simulink model "a2024_V2X_6V_Simulink_model"  (R2023b)
settings: Solver=VariableStepAuto  StartTime=0.0  StopTime=30  MaxStep=1e-2  RelTol=1e-3  AbsTol=1e-3
values from neighbouring files (symbols this model uses):
  b = 1.6    [a2024_v2x_matlab_6veh.m]
  mEgo = 1500    [a2024_v2x_matlab_6veh.m]
  Mode = 1    [a2024_v2x_matlab_6veh.m]    (also in v2x_matlab.m; v2x_matlabV2.m; v2x_matlab_6veh.m; v2x_matlab_R.m)
  pilot = (randi(s,[0 1],pilotsPerSym,1)-0.5)*2    [v2x_matlab.m]
  RxPowerV1 = zeros(sizeEgoWP+2, sizeV1WP+2)    [a2024_v2x_matlab_6veh.m]
  RxPowerV2 = zeros(sizeEgoWP+2, sizeV2WP+2)    [a2024_v2x_matlab_6veh.m]
  RxPowerV3 = zeros(sizeEgoWP+2, sizeV3WP+2)    [a2024_v2x_matlab_6veh.m]
  RxPowerV4 = zeros(sizeEgoWP+2, sizeV4WP+2)    [a2024_v2x_matlab_6veh.m]
  RxPowerV5 = zeros(sizeEgoWP+2, sizeV5WP+2)    [a2024_v2x_matlab_6veh.m]
  RxPowerV6 = zeros(sizeEgoWP+2, sizeV6WP+2)    [a2024_v2x_matlab_6veh.m]
  sampleTime = 0.1    [a2024_v2x_matlab_6veh.m]    (also in v2x_matlab.m; v2x_matlabV2.m; v2x_matlab_6veh.m; v2x_matlab_R.m)
  t_gap = 1.4    [a2024_v2x_matlab_6veh.m]
  waypoints = [egoWP(:,2) egoWP(:,1), zeroforwp]    [a2024_v2x_matlab_6veh.m]    (also in misc.m = data.data.ActorSpecifications(1,1).Waypoints(:,[1,2]); v2x_matlab.m = data.data.ActorSpecifications(1,1).Waypoints(:,[1,2]); v2x_matlabV2.m = [5 -1.6 0; v2x_matlab_R.m = [5 -1.6 0)
  ZeroActors = struct(     'ActorID',0,     'Position', [1000 1000 1000],      'Velocity', [0 0 0],      'Roll', 0,      'Pitch', 0,      'Yaw', 0,      'AngularVelocity', [0 0 0])    [v2x_matlabV2.m]    (also in v2x_matlab_R.m)
undefined symbols (not defined in the file or in its folder): driving, PredictionHorizon, Ts
libraries: commofdm x50, commcnvcod2 x39, simulink x34, commdigbbndam3 x31, commblkintrlv2 x26, commdigbbndpm3 x14, simulink_extras x12, drivingscenarioandsensors x3, mpcadaslib x2, commchan3 x1, vehdynlibdriver x1, commrandsrc3 x1
(part 2 of 6)

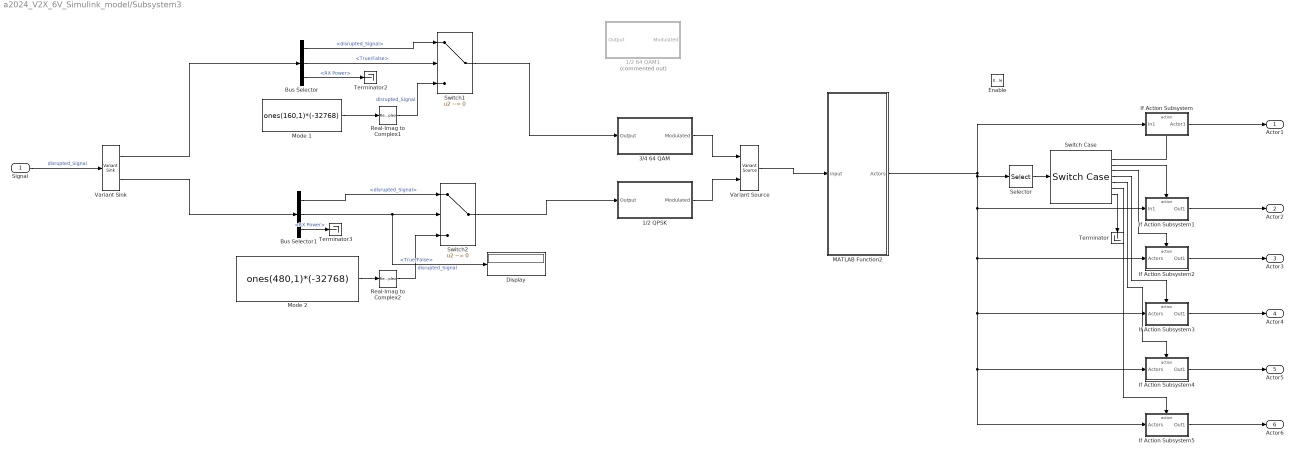
== system a2024_V2X_6V_Simulink_model/Subsystem3 ==
  Signal : Inport
  Enable : EnablePort
  1/2 64 QAM1 : Subsystem  Commented=on  TreatAsAtomicUnit=on
  1/2 QPSK : Subsystem  TreatAsAtomicUnit=on
  3/4 64 QAM : Subsystem  TreatAsAtomicUnit=on
  Bus Selector : BusSelector  OutputSignals=disrupted_Signal,True/False,RX Power
  Bus Selector1 : BusSelector  OutputSignals=disrupted_Signal,True/False,RX Power
  Display : Display
  If Action Subsystem : Subsystem  TreatAsAtomicUnit=on
  If Action Subsystem1 : Subsystem  TreatAsAtomicUnit=on
  If Action Subsystem2 : Subsystem  TreatAsAtomicUnit=on
  If Action Subsystem3 : Subsystem  TreatAsAtomicUnit=on
  If Action Subsystem4 : Subsystem  TreatAsAtomicUnit=on
  If Action Subsystem5 : Subsystem  TreatAsAtomicUnit=on
  MATLAB Function2 : MATLAB Function  TreatAsAtomicUnit=on  SystemSampleTime=0.01
  Mode 1 : Constant  Value=ones(160,1)*(-32768)  OutDataTypeStr=Inherit: Inherit via back propagation
  Mode 2 : Constant  Value=ones(480,1)*(-32768)  OutDataTypeStr=Inherit: Inherit via back propagation
  Real-Imag to Complex1 : RealImagToComplex  Input=Real
  Real-Imag to Complex2 : RealImagToComplex  Input=Real
  Selector : Selector  IndexOptions=Index vector (dialog)  Indices=[3]  OutputSizes=1
  Switch Case : SwitchCase  CaseConditions={1,2,3,4,5,6}
  Switch1 : Switch  Criteria=u2 ~= 0  OutDataTypeStr=double  SaturateOnIntegerOverflow=off  InputSameDT=off
  Switch2 : Switch  Criteria=u2 ~= 0  OutDataTypeStr=double  SaturateOnIntegerOverflow=off  InputSameDT=off
  Terminator : Terminator
  Terminator2 : Terminator
  Terminator3 : Terminator
  Variant Sink : VariantSink
  Variant Source : VariantSource
  Actor1 : Outport
  Actor2 : Outport  Port=2
  Actor3 : Outport  Port=3
  Actor4 : Outport  Port=4
  Actor5 : Outport  Port=5
  Actor6 : Outport  Port=6
  wires:
  Selector/1 -> Switch Case/1
  Switch Case/1 -> If Action Subsystem/Action
  If Action Subsystem/1(Actor1) -> Actor1/1
  If Action Subsystem1/1(Out1) -> Actor2/1
  Switch Case/2 -> If Action Subsystem1/Action
  If Action Subsystem2/1(Out1) -> Actor3/1
  Switch Case/3 -> If Action Subsystem2/Action
  If Action Subsystem3/1(Out1) -> Actor4/1
  MATLAB Function2/1(Actors) -> If Action Subsystem5/1(Actors), If Action Subsystem4/1(Actors), If Action Subsystem3/1(Actors), If Action Subsystem2/1(Actors), If Action Subsystem1/1(In1), Selector/1, If Action Subsystem/1(In1)
  Switch Case/4 -> If Action Subsystem3/Action
  Switch Case/7 -> Terminator/1
  If Action Subsystem4/1(Out1) -> Actor5/1
  Switch Case/5 -> If Action Subsystem4/Action
  If Action Subsystem5/1(Out1) -> Actor6/1
  Switch Case/6 -> If Action Subsystem5/Action
  3/4 64 QAM/1(Modulated) -> Variant Source/1
  1/2 QPSK/1(Modulated) -> Variant Source/2
  Variant Source/1 -> MATLAB Function2/1(input)
  Switch1/1 -> 3/4 64 QAM/1(Output)
  Switch2/1 -> 1/2 QPSK/1(Output)
  Signal/1 -> Variant Sink/1  "disrupted_Signal"
  Variant Sink/1 -> Bus Selector/1
  Variant Sink/2 -> Bus Selector1/1
  Bus Selector/1 -> Switch1/1  "<disrupted_Signal>"
  Bus Selector/3 -> Terminator2/1  "<RX Power>"
  Bus Selector/2 -> Switch1/2  "<True/False>"
  Mode 1/1 -> Real-Imag to Complex1/1
  Real-Imag to Complex1/1 -> Switch1/3  "disrupted_Signal"
  Mode 2/1 -> Real-Imag to Complex2/1
  Bus Selector1/1 -> Switch2/1  "<disrupted_Signal>"
  Real-Imag to Complex2/1 -> Switch2/3  "disrupted_Signal"
  Bus Selector1/2 -> Display/1, Switch2/2  "<True/False>"
  Bus Selector1/3 -> Terminator3/1  "<RX Power>"

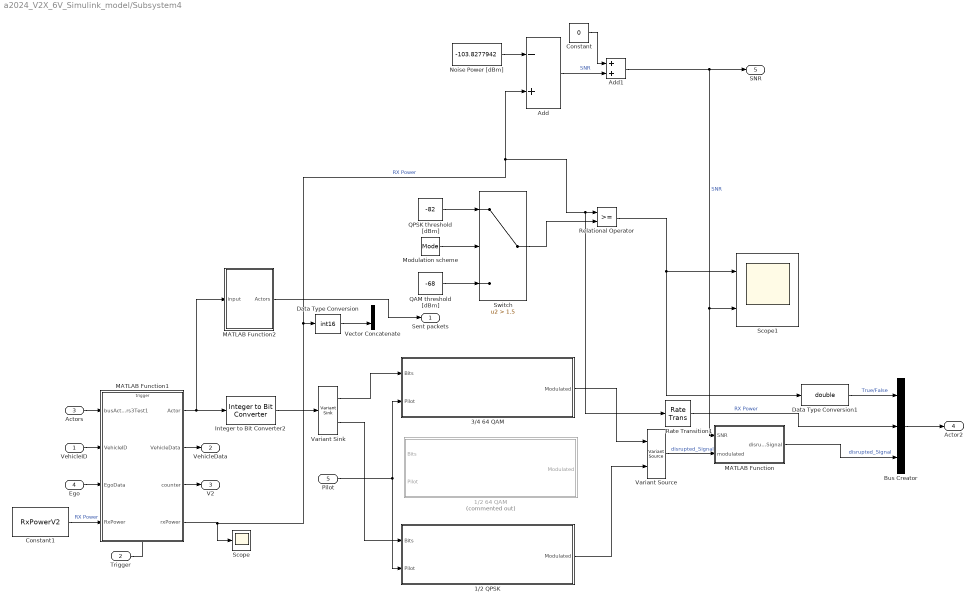
== system a2024_V2X_6V_Simulink_model/Subsystem4 ==
  VehicleID : Inport
  Trigger : Inport  Port=2
  Actors : Inport  Port=3
  Ego : Inport  Port=4
  Pilot : Inport  Port=5
  1/2 64 QAM : Subsystem  Commented=on  TreatAsAtomicUnit=on
  1/2 QPSK : Subsystem  TreatAsAtomicUnit=on
  3/4 64 QAM : Subsystem  TreatAsAtomicUnit=on
  Add : Sum  Inputs=-+
  Add1 : Sum
  Bus Creator : BusCreator  Inputs=3
  Constant : Constant  Value=0
  Constant1 : Constant  Value=RxPowerV2
  Data Type Conversion : DataTypeConversion  OutDataTypeStr=int16  SaturateOnIntegerOverflow=off  RndMeth=Floor
  Data Type Conversion1 : DataTypeConversion  OutDataTypeStr=double  SaturateOnIntegerOverflow=off  RndMeth=Floor
  Integer to Bit Converter2 : simulink/Logic and Bit Operations/Integer to Bit Converter  nbits=16  signedInputValues=Signed  bitOrder=MSB first  outDtype=boolean
  MATLAB Function : MATLAB Function  TreatAsAtomicUnit=on
  MATLAB Function1 : MATLAB Function  TreatAsAtomicUnit=on
  MATLAB Function2 : MATLAB Function  TreatAsAtomicUnit=on  SystemSampleTime=0.01
  Modulation scheme : Constant  Value=Mode
  Noise Power [dBm] : Constant  Value=-103.8277942
  QAM threshold [dBm] : Constant  Value=-68
  QPSK threshold [dBm] : Constant  Value=-82
  Rate Transition1 : RateTransition  OutPortSampleTime=sampleTime/10
  Relational Operator : RelationalOperator  OutDataTypeStr=boolean  RndMeth=Simplest  InputSameDT=off
  Scope : Scope
  Scope1 : Scope  NumInputPorts=2
  Switch : Switch  Criteria=u2 > Threshold  Threshold=1.5  SaturateOnIntegerOverflow=off  InputSameDT=off
  Variant Sink : VariantSink
  Variant Source : VariantSource
  Vector Concatenate : Concatenate
  Sent packets : Outport
  VehicleData : Outport  Port=2
  V2 : Outport  Port=3
  Actor2 : Outport  Port=4
  SNR : Outport  Port=5
  wires:
  Constant/1 -> Add1/1
  Add/1 -> Add1/2  "SNR"
  Variant Source/1 -> MATLAB Function/2(modulated)  "disrupted_Signal"
  Rate Transition1/1 -> Bus Creator/2  "RX Power"
  Data Type Conversion1/1 -> Bus Creator/1  "True/False"
  Data Type Conversion/1 -> Vector Concatenate/2
  MATLAB Function/1(disrupted_Signal) -> Bus Creator/3  "disrupted_Signal"
  MATLAB Function2/1(Actors) -> Sent packets/1
  Bus Creator/1 -> Actor2/1
  Constant1/1 -> MATLAB Function1/4(RxPower)  "RX Power"
  MATLAB Function1/4(rxPower) -> Add/2, Relational Operator/1, Rate Transition1/1, Data Type Conversion/1, Scope/1  "RX Power"
  Relational Operator/1 -> Scope1/1, Data Type Conversion1/1
  Switch/1 -> Relational Operator/2
  Add1/1 -> SNR/1, Scope1/2, MATLAB Function/1(SNR)  "SNR"
  Modulation scheme/1 -> Switch/2
  QAM threshold [dBm]/1 -> Switch/3
  QPSK threshold [dBm]/1 -> Switch/1
  Noise Power [dBm]/1 -> Add/1
  Variant Sink/2 -> 1/2 QPSK/1(Bits)
  Variant Sink/1 -> 3/4 64 QAM/1(Bits)
  1/2 QPSK/1(Modulated) -> Variant Source/2
  3/4 64 QAM/1(Modulated) -> Variant Source/1
  Pilot/1 -> 3/4 64 QAM/2(Pilot), 1/2 QPSK/2(Pilot)
  Integer to Bit Converter2/1 -> Variant Sink/1
  Trigger/1 -> MATLAB Function1/Trigger
  MATLAB Function1/3(counter) -> V2/1
  MATLAB Function1/2(VehicleData) -> VehicleData/1
  VehicleID/1 -> MATLAB Function1/2(VehicleID)
  Actors/1 -> MATLAB Function1/1(busActors3Test1)
  Ego/1 -> MATLAB Function1/3(EgoData)
  MATLAB Function1/1(Actor) -> Integer to Bit Converter2/1, MATLAB Function2/1(input)

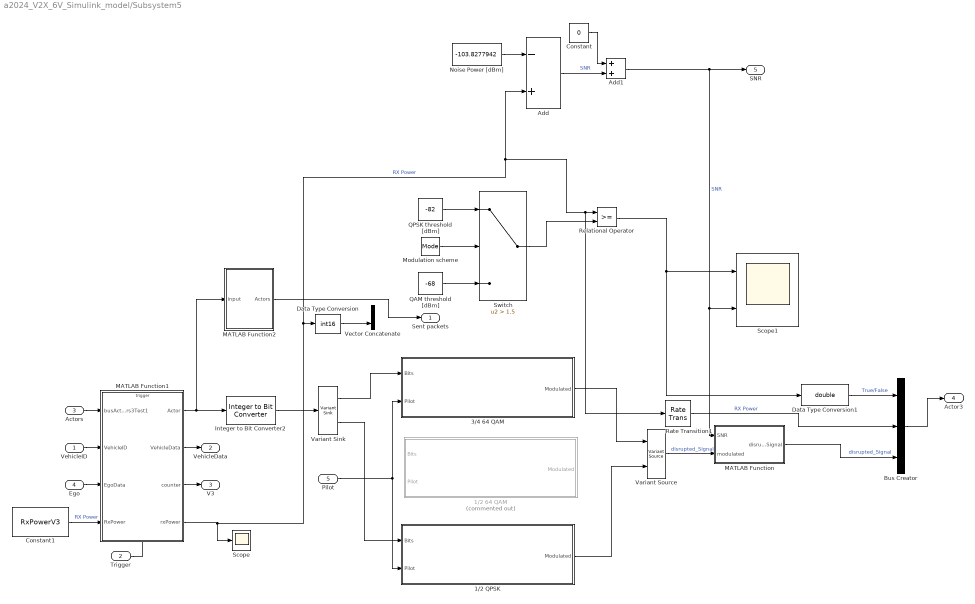
== system a2024_V2X_6V_Simulink_model/Subsystem5 ==
  VehicleID : Inport
  Trigger : Inport  Port=2
  Actors : Inport  Port=3
  Ego : Inport  Port=4
  Pilot : Inport  Port=5
  1/2 64 QAM : Subsystem  Commented=on  TreatAsAtomicUnit=on
  1/2 QPSK : Subsystem  TreatAsAtomicUnit=on
  3/4 64 QAM : Subsystem  TreatAsAtomicUnit=on
  Add : Sum  Inputs=-+
  Add1 : Sum
  Bus Creator : BusCreator  Inputs=3
  Constant : Constant  Value=0
  Constant1 : Constant  Value=RxPowerV3
  Data Type Conversion : DataTypeConversion  OutDataTypeStr=int16  SaturateOnIntegerOverflow=off  RndMeth=Floor
  Data Type Conversion1 : DataTypeConversion  OutDataTypeStr=double  SaturateOnIntegerOverflow=off  RndMeth=Floor
  Integer to Bit Converter2 : simulink/Logic and Bit Operations/Integer to Bit Converter  nbits=16  signedInputValues=Signed  bitOrder=MSB first  outDtype=boolean
  MATLAB Function : MATLAB Function  TreatAsAtomicUnit=on
  MATLAB Function1 : MATLAB Function  TreatAsAtomicUnit=on
  MATLAB Function2 : MATLAB Function  TreatAsAtomicUnit=on  SystemSampleTime=0.01
  Modulation scheme : Constant  Value=Mode
  Noise Power [dBm] : Constant  Value=-103.8277942
  QAM threshold [dBm] : Constant  Value=-68
  QPSK threshold [dBm] : Constant  Value=-82
  Rate Transition1 : RateTransition  OutPortSampleTime=sampleTime/10
  Relational Operator : RelationalOperator  OutDataTypeStr=boolean  RndMeth=Simplest  InputSameDT=off
  Scope : Scope
  Scope1 : Scope  NumInputPorts=2
  Switch : Switch  Criteria=u2 > Threshold  Threshold=1.5  SaturateOnIntegerOverflow=off  InputSameDT=off
  Variant Sink : VariantSink
  Variant Source : VariantSource
  Vector Concatenate : Concatenate
  Sent packets : Outport
  VehicleData : Outport  Port=2
  V3 : Outport  Port=3
  Actor3 : Outport  Port=4
  SNR : Outport  Port=5
  wires:
  MATLAB Function1/1(Actor) -> MATLAB Function2/1(input), Integer to Bit Converter2/1
  Ego/1 -> MATLAB Function1/3(EgoData)
  Actors/1 -> MATLAB Function1/1(busActors3Test1)
  VehicleID/1 -> MATLAB Function1/2(VehicleID)
  MATLAB Function1/2(VehicleData) -> VehicleData/1
  MATLAB Function1/3(counter) -> V3/1
  Trigger/1 -> MATLAB Function1/Trigger
  Integer to Bit Converter2/1 -> Variant Sink/1
  Pilot/1 -> 1/2 QPSK/2(Pilot), 3/4 64 QAM/2(Pilot)
  3/4 64 QAM/1(Modulated) -> Variant Source/1
  1/2 QPSK/1(Modulated) -> Variant Source/2
  Variant Sink/1 -> 3/4 64 QAM/1(Bits)
  Variant Sink/2 -> 1/2 QPSK/1(Bits)
  Noise Power [dBm]/1 -> Add/1
  QPSK threshold [dBm]/1 -> Switch/1
  QAM threshold [dBm]/1 -> Switch/3
  Modulation scheme/1 -> Switch/2
  Add1/1 -> MATLAB Function/1(SNR), Scope1/2, SNR/1  "SNR"
  Switch/1 -> Relational Operator/2
  Relational Operator/1 -> Data Type Conversion1/1, Scope1/1
  MATLAB Function1/4(rxPower) -> Scope/1, Data Type Conversion/1, Rate Transition1/1, Relational Operator/1, Add/2  "RX Power"
  Constant1/1 -> MATLAB Function1/4(RxPower)  "RX Power"
  Bus Creator/1 -> Actor3/1
  MATLAB Function2/1(Actors) -> Sent packets/1
  MATLAB Function/1(disrupted_Signal) -> Bus Creator/3  "disrupted_Signal"
  Data Type Conversion/1 -> Vector Concatenate/2
  Data Type Conversion1/1 -> Bus Creator/1  "True/False"
  Rate Transition1/1 -> Bus Creator/2  "RX Power"
  Variant Source/1 -> MATLAB Function/2(modulated)  "disrupted_Signal"
  Add/1 -> Add1/2  "SNR"
  Constant/1 -> Add1/1

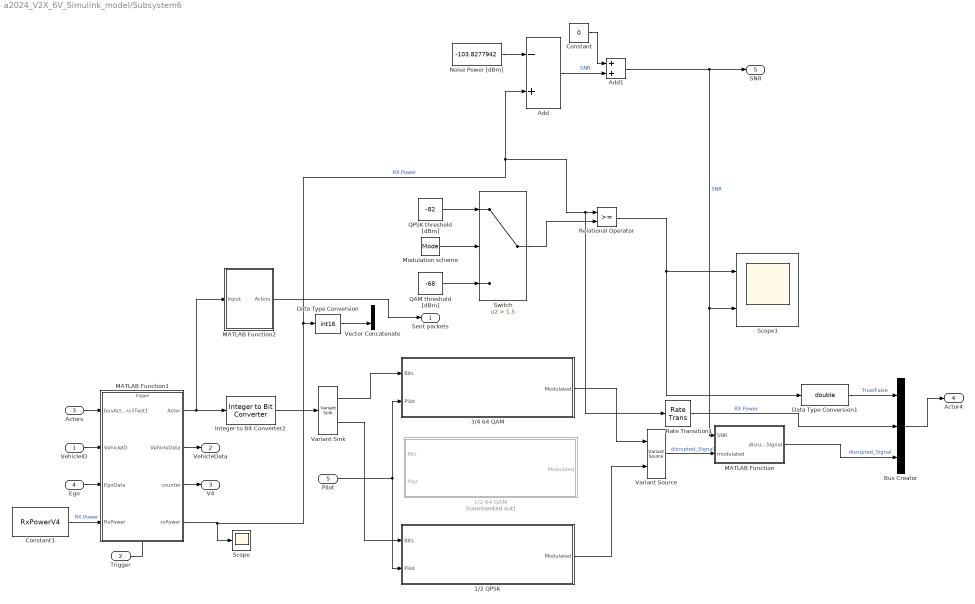
== system a2024_V2X_6V_Simulink_model/Subsystem6 ==
  VehicleID : Inport
  Trigger : Inport  Port=2
  Actors : Inport  Port=3
  Ego : Inport  Port=4
  Pilot : Inport  Port=5
  1/2 64 QAM : Subsystem  Commented=on  TreatAsAtomicUnit=on
  1/2 QPSK : Subsystem  TreatAsAtomicUnit=on
  3/4 64 QAM : Subsystem  TreatAsAtomicUnit=on
  Add : Sum  Inputs=-+
  Add1 : Sum
  Bus Creator : BusCreator  Inputs=3
  Constant : Constant  Value=0
  Constant1 : Constant  Value=RxPowerV4
  Data Type Conversion : DataTypeConversion  OutDataTypeStr=int16  SaturateOnIntegerOverflow=off  RndMeth=Floor
  Data Type Conversion1 : DataTypeConversion  OutDataTypeStr=double  SaturateOnIntegerOverflow=off  RndMeth=Floor
  Integer to Bit Converter2 : simulink/Logic and Bit Operations/Integer to Bit Converter  nbits=16  signedInputValues=Signed  bitOrder=MSB first  outDtype=boolean
  MATLAB Function : MATLAB Function  TreatAsAtomicUnit=on
  MATLAB Function1 : MATLAB Function  TreatAsAtomicUnit=on
  MATLAB Function2 : MATLAB Function  TreatAsAtomicUnit=on  SystemSampleTime=0.01
  Modulation scheme : Constant  Value=Mode
  Noise Power [dBm] : Constant  Value=-103.8277942
  QAM threshold [dBm] : Constant  Value=-68
  QPSK threshold [dBm] : Constant  Value=-82
  Rate Transition1 : RateTransition  OutPortSampleTime=sampleTime/10
  Relational Operator : RelationalOperator  OutDataTypeStr=boolean  RndMeth=Simplest  InputSameDT=off
  Scope : Scope
  Scope1 : Scope  NumInputPorts=2
  Switch : Switch  Criteria=u2 > Threshold  Threshold=1.5  SaturateOnIntegerOverflow=off  InputSameDT=off
  Variant Sink : VariantSink
  Variant Source : VariantSource
  Vector Concatenate : Concatenate
  Sent packets : Outport
  VehicleData : Outport  Port=2
  V4 : Outport  Port=3
  Actor4 : Outport  Port=4
  SNR : Outport  Port=5
  wires:
  Constant/1 -> Add1/1
  Add/1 -> Add1/2  "SNR"
  Variant Source/1 -> MATLAB Function/2(modulated)  "disrupted_Signal"
  Rate Transition1/1 -> Bus Creator/2  "RX Power"
  Data Type Conversion1/1 -> Bus Creator/1  "True/False"
  Data Type Conversion/1 -> Vector Concatenate/2
  MATLAB Function/1(disrupted_Signal) -> Bus Creator/3  "disrupted_Signal"
  MATLAB Function2/1(Actors) -> Sent packets/1
  Bus Creator/1 -> Actor4/1
  Constant1/1 -> MATLAB Function1/4(RxPower)  "RX Power"
  MATLAB Function1/4(rxPower) -> Add/2, Relational Operator/1, Rate Transition1/1, Data Type Conversion/1, Scope/1  "RX Power"
  Relational Operator/1 -> Scope1/1, Data Type Conversion1/1
  Switch/1 -> Relational Operator/2
  Add1/1 -> SNR/1, Scope1/2, MATLAB Function/1(SNR)  "SNR"
  Modulation scheme/1 -> Switch/2
  QAM threshold [dBm]/1 -> Switch/3
  QPSK threshold [dBm]/1 -> Switch/1
  Noise Power [dBm]/1 -> Add/1
  Variant Sink/2 -> 1/2 QPSK/1(Bits)
  Variant Sink/1 -> 3/4 64 QAM/1(Bits)
  1/2 QPSK/1(Modulated) -> Variant Source/2
  3/4 64 QAM/1(Modulated) -> Variant Source/1
  Pilot/1 -> 3/4 64 QAM/2(Pilot), 1/2 QPSK/2(Pilot)
  Integer to Bit Converter2/1 -> Variant Sink/1
  Trigger/1 -> MATLAB Function1/Trigger
  MATLAB Function1/3(counter) -> V4/1
  MATLAB Function1/2(VehicleData) -> VehicleData/1
  VehicleID/1 -> MATLAB Function1/2(VehicleID)
  Actors/1 -> MATLAB Function1/1(busActors3Test1)
  Ego/1 -> MATLAB Function1/3(EgoData)
  MATLAB Function1/1(Actor) -> Integer to Bit Converter2/1, MATLAB Function2/1(input)

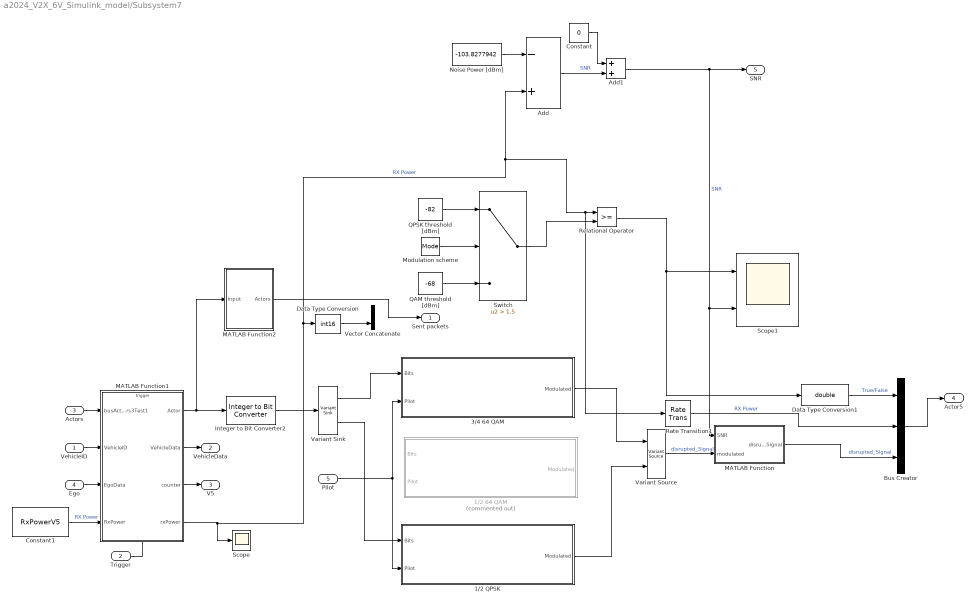
== system a2024_V2X_6V_Simulink_model/Subsystem7 ==
  VehicleID : Inport
  Trigger : Inport  Port=2
  Actors : Inport  Port=3
  Ego : Inport  Port=4
  Pilot : Inport  Port=5
  1/2 64 QAM : Subsystem  Commented=on  TreatAsAtomicUnit=on
  1/2 QPSK : Subsystem  TreatAsAtomicUnit=on
  3/4 64 QAM : Subsystem  TreatAsAtomicUnit=on
  Add : Sum  Inputs=-+
  Add1 : Sum
  Bus Creator : BusCreator  Inputs=3
  Constant : Constant  Value=0
  Constant1 : Constant  Value=RxPowerV5
  Data Type Conversion : DataTypeConversion  OutDataTypeStr=int16  SaturateOnIntegerOverflow=off  RndMeth=Floor
  Data Type Conversion1 : DataTypeConversion  OutDataTypeStr=double  SaturateOnIntegerOverflow=off  RndMeth=Floor
  Integer to Bit Converter2 : simulink/Logic and Bit Operations/Integer to Bit Converter  nbits=16  signedInputValues=Signed  bitOrder=MSB first  outDtype=boolean
  MATLAB Function : MATLAB Function  TreatAsAtomicUnit=on
  MATLAB Function1 : MATLAB Function  TreatAsAtomicUnit=on
  MATLAB Function2 : MATLAB Function  TreatAsAtomicUnit=on  SystemSampleTime=0.01
  Modulation scheme : Constant  Value=Mode
  Noise Power [dBm] : Constant  Value=-103.8277942
  QAM threshold [dBm] : Constant  Value=-68
  QPSK threshold [dBm] : Constant  Value=-82
  Rate Transition1 : RateTransition  OutPortSampleTime=sampleTime/10
  Relational Operator : RelationalOperator  OutDataTypeStr=boolean  RndMeth=Simplest  InputSameDT=off
  Scope : Scope
  Scope1 : Scope  NumInputPorts=2
  Switch : Switch  Criteria=u2 > Threshold  Threshold=1.5  SaturateOnIntegerOverflow=off  InputSameDT=off
  Variant Sink : VariantSink
  Variant Source : VariantSource
  Vector Concatenate : Concatenate
  Sent packets : Outport
  VehicleData : Outport  Port=2
  V5 : Outport  Port=3
  Actor5 : Outport  Port=4
  SNR : Outport  Port=5
  wires:
  MATLAB Function1/1(Actor) -> MATLAB Function2/1(input), Integer to Bit Converter2/1
  Ego/1 -> MATLAB Function1/3(EgoData)
  Actors/1 -> MATLAB Function1/1(busActors3Test1)
  VehicleID/1 -> MATLAB Function1/2(VehicleID)
  MATLAB Function1/2(VehicleData) -> VehicleData/1
  MATLAB Function1/3(counter) -> V5/1
  Trigger/1 -> MATLAB Function1/Trigger
  Integer to Bit Converter2/1 -> Variant Sink/1
  Pilot/1 -> 1/2 QPSK/2(Pilot), 3/4 64 QAM/2(Pilot)
  3/4 64 QAM/1(Modulated) -> Variant Source/1
  1/2 QPSK/1(Modulated) -> Variant Source/2
  Variant Sink/1 -> 3/4 64 QAM/1(Bits)
  Variant Sink/2 -> 1/2 QPSK/1(Bits)
  Noise Power [dBm]/1 -> Add/1
  QPSK threshold [dBm]/1 -> Switch/1
  QAM threshold [dBm]/1 -> Switch/3
  Modulation scheme/1 -> Switch/2
  Add1/1 -> MATLAB Function/1(SNR), Scope1/2, SNR/1  "SNR"
  Switch/1 -> Relational Operator/2
  Relational Operator/1 -> Data Type Conversion1/1, Scope1/1
  MATLAB Function1/4(rxPower) -> Scope/1, Data Type Conversion/1, Rate Transition1/1, Relational Operator/1, Add/2  "RX Power"
  Constant1/1 -> MATLAB Function1/4(RxPower)  "RX Power"
  Bus Creator/1 -> Actor5/1
  MATLAB Function2/1(Actors) -> Sent packets/1
  MATLAB Function/1(disrupted_Signal) -> Bus Creator/3  "disrupted_Signal"
  Data Type Conversion/1 -> Vector Concatenate/2
  Data Type Conversion1/1 -> Bus Creator/1  "True/False"
  Rate Transition1/1 -> Bus Creator/2  "RX Power"
  Variant Source/1 -> MATLAB Function/2(modulated)  "disrupted_Signal"
  Add/1 -> Add1/2  "SNR"
  Constant/1 -> Add1/1

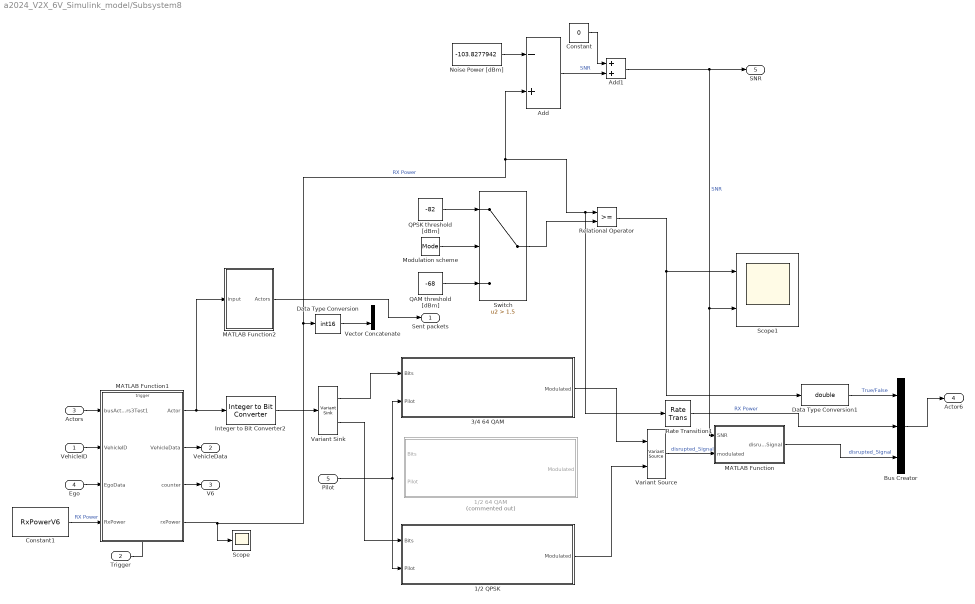
== system a2024_V2X_6V_Simulink_model/Subsystem8 ==
  VehicleID : Inport
  Trigger : Inport  Port=2
  Actors : Inport  Port=3
  Ego : Inport  Port=4
  Pilot : Inport  Port=5
  1/2 64 QAM : Subsystem  Commented=on  TreatAsAtomicUnit=on
  1/2 QPSK : Subsystem  TreatAsAtomicUnit=on
  3/4 64 QAM : Subsystem  TreatAsAtomicUnit=on
  Add : Sum  Inputs=-+
  Add1 : Sum
  Bus Creator : BusCreator  Inputs=3
  Constant : Constant  Value=0
  Constant1 : Constant  Value=RxPowerV6
  Data Type Conversion : DataTypeConversion  OutDataTypeStr=int16  SaturateOnIntegerOverflow=off  RndMeth=Floor
  Data Type Conversion1 : DataTypeConversion  OutDataTypeStr=double  SaturateOnIntegerOverflow=off  RndMeth=Floor
  Integer to Bit Converter2 : simulink/Logic and Bit Operations/Integer to Bit Converter  nbits=16  signedInputValues=Signed  bitOrder=MSB first  outDtype=boolean
  MATLAB Function : MATLAB Function  TreatAsAtomicUnit=on
  MATLAB Function1 : MATLAB Function  TreatAsAtomicUnit=on
  MATLAB Function2 : MATLAB Function  TreatAsAtomicUnit=on  SystemSampleTime=0.01
  Modulation scheme : Constant  Value=Mode
  Noise Power [dBm] : Constant  Value=-103.8277942
  QAM threshold [dBm] : Constant  Value=-68
  QPSK threshold [dBm] : Constant  Value=-82
  Rate Transition1 : RateTransition  OutPortSampleTime=sampleTime/10
  Relational Operator : RelationalOperator  OutDataTypeStr=boolean  RndMeth=Simplest  InputSameDT=off
  Scope : Scope
  Scope1 : Scope  NumInputPorts=2
  Switch : Switch  Criteria=u2 > Threshold  Threshold=1.5  SaturateOnIntegerOverflow=off  InputSameDT=off
  Variant Sink : VariantSink
  Variant Source : VariantSource
  Vector Concatenate : Concatenate
  Sent packets : Outport
  VehicleData : Outport  Port=2
  V6 : Outport  Port=3
  Actor6 : Outport  Port=4
  SNR : Outport  Port=5
  wires:
  Constant/1 -> Add1/1
  Add/1 -> Add1/2  "SNR"
  Variant Source/1 -> MATLAB Function/2(modulated)  "disrupted_Signal"
  Rate Transition1/1 -> Bus Creator/2  "RX Power"
  Data Type Conversion1/1 -> Bus Creator/1  "True/False"
  Data Type Conversion/1 -> Vector Concatenate/2
  MATLAB Function/1(disrupted_Signal) -> Bus Creator/3  "disrupted_Signal"
  MATLAB Function2/1(Actors) -> Sent packets/1
  Bus Creator/1 -> Actor6/1
  Constant1/1 -> MATLAB Function1/4(RxPower)  "RX Power"
  MATLAB Function1/4(rxPower) -> Add/2, Relational Operator/1, Rate Transition1/1, Data Type Conversion/1, Scope/1  "RX Power"
  Relational Operator/1 -> Scope1/1, Data Type Conversion1/1
  Switch/1 -> Relational Operator/2
  Add1/1 -> SNR/1, Scope1/2, MATLAB Function/1(SNR)  "SNR"
  Modulation scheme/1 -> Switch/2
  QAM threshold [dBm]/1 -> Switch/3
  QPSK threshold [dBm]/1 -> Switch/1
  Noise Power [dBm]/1 -> Add/1
  Variant Sink/2 -> 1/2 QPSK/1(Bits)
  Variant Sink/1 -> 3/4 64 QAM/1(Bits)
  1/2 QPSK/1(Modulated) -> Variant Source/2
  3/4 64 QAM/1(Modulated) -> Variant Source/1
  Pilot/1 -> 3/4 64 QAM/2(Pilot), 1/2 QPSK/2(Pilot)
  Integer to Bit Converter2/1 -> Variant Sink/1
  Trigger/1 -> MATLAB Function1/Trigger
  MATLAB Function1/3(counter) -> V6/1
  MATLAB Function1/2(VehicleData) -> VehicleData/1
  VehicleID/1 -> MATLAB Function1/2(VehicleID)
  Actors/1 -> MATLAB Function1/1(busActors3Test1)
  Ego/1 -> MATLAB Function1/3(EgoData)
  MATLAB Function1/1(Actor) -> Integer to Bit Converter2/1, MATLAB Function2/1(input)

== system a2024_V2X_6V_Simulink_model/Subsystem9 ==
  Inport : Inport
  1/2 64 QAM1 : Subsystem  Commented=on  TreatAsAtomicUnit=on
  1/2 QPSK : Subsystem  TreatAsAtomicUnit=on
  3/4 64 QAM : Subsystem  TreatAsAtomicUnit=on
  Bus Selector6 : BusSelector  OutputSignals=disrupted_Signal,True/False,RX Power
  Bus Selector7 : BusSelector  OutputSignals=disrupted_Signal,True/False,RX Power
  Display : Display
  MATLAB Function2 : MATLAB Function  TreatAsAtomicUnit=on  SystemSampleTime=0.01
  Mode 1 : Constant  Value=ones(160,1)*(-32768)  OutDataTypeStr=Inherit: Inherit via back propagation
  Mode 2 : Constant  Value=ones(480,1)*(-32768)  OutDataTypeStr=Inherit: Inherit via back propagation
  Real-Imag to Complex1 : RealImagToComplex  Input=Real
  Real-Imag to Complex2 : RealImagToComplex  Input=Real
  Switch1 : Switch  Criteria=u2 ~= 0  OutDataTypeStr=double  SaturateOnIntegerOverflow=off  InputSameDT=off
  Switch2 : Switch  Criteria=u2 ~= 0  OutDataTypeStr=double  SaturateOnIntegerOverflow=off  InputSameDT=off
  Terminator2 : Terminator
  Terminator3 : Terminator
  Variant Sink : VariantSink
  Variant Source : VariantSource
  Outport : Outport
  wires:
  Real-Imag to Complex1/1 -> Switch1/3  "disrupted_Signal"
  Variant Source/1 -> MATLAB Function2/1(input)
  Bus Selector6/1 -> Switch1/1  "<disrupted_Signal>"
  1/2 QPSK/1(Modulated) -> Variant Source/2
  Inport/1 -> Variant Sink/1
  MATLAB Function2/1(Actors) -> Outport/1
  Variant Sink/1 -> Bus Selector6/1
  Real-Imag to Complex2/1 -> Switch2/3  "disrupted_Signal"
  Variant Sink/2 -> Bus Selector7/1
  Mode 2/1 -> Real-Imag to Complex2/1
  Bus Selector6/2 -> Switch1/2  "<True/False>"
  Bus Selector6/3 -> Terminator2/1  "<RX Power>"
  3/4 64 QAM/1(Modulated) -> Variant Source/1
  Bus Selector7/2 -> Display/1, Switch2/2  "<True/False>"
  Switch1/1 -> 3/4 64 QAM/1(Output)
  Bus Selector7/3 -> Terminator3/1  "<RX Power>"
  Switch2/1 -> 1/2 QPSK/1(Output)
  Bus Selector7/1 -> Switch2/1  "<disrupted_Signal>"
  Mode 1/1 -> Real-Imag to Complex1/1

== system a2024_V2X_6V_Simulink_model/Vehicle 2 ==
  trigger : Inport
  VehicleID : Inport  Port=2
  Pilot : Inport  Port=3
  busActors3Test1 : Inport  Port=4
  Constant2 : Constant  Value=[zeros(19,1)']  SampleTime=-1
  Entity Multicast1 : EntityMulticast  InputPortMessageModes=m
  Integer to Bit Converter1 : simulink/Logic and Bit Operations/Integer to Bit Converter  nbits=16  signedInputValues=Signed  bitOrder=MSB first  outDtype=boolean
  MATLAB Function1 : MATLAB Function  TreatAsAtomicUnit=on
  OFDM Modulator1 : commofdm/OFDM Modulator  StatePerturbationForJacobian=1.0e-05  FFTLength=64  NumGuardBandCarriers=[0;0]  InsertDCNull=on  PilotInputPort=on  PilotCarrierIndices=[12; 26; 40; 54]  CyclicPrefixLength=32  Windowing=off  WindowLength=16  OversamplingFactor=3  NumSymbols=1  NumTransmitAntennas=1  SimulateUsing=Interpreted execution
  Rectangular QAM Modulator Baseband1 : commdigbbndam3/Rectangular QAM Modulator Baseband  M=2^6  InType=Bit  Enc=Binary  Mapping=[0:15]  PowType=Average Power  MinDist=2  AvgPow=P_Signal  PeakPow=1  Ph=0  outDtype=double  outWordLen=16  outUDDataType=sfix(16)  outFracLenMode=Best precision  outFracLen=15  outDataTypeStr=double  outLastDataTypeStr=double
      settings: LibrarySourceBlock=|
      | commhdldigbbndam/Rectangular QAM
      | Modulator
      | Baseband
  Send1 : Send  OutputPortMessageModes=m
  Vector Concatenate1 : Concatenate
  wires:
  busActors3Test1/1 -> MATLAB Function1/1(busActors3Test1)
  Rectangular QAM Modulator Baseband1/1 -> Vector Concatenate1/1
  Constant2/1 -> Vector Concatenate1/2
  Send1/1 -> Entity Multicast1/1
  Integer to Bit Converter1/1 -> Rectangular QAM Modulator Baseband1/1
  Vector Concatenate1/1 -> OFDM Modulator1/1  "After QAM Mod"
  OFDM Modulator1/1 -> Send1/1  "OFDM modulated"
  MATLAB Function1/1(intVector) -> Integer to Bit Converter1/1
  trigger/1 -> MATLAB Function1/Trigger
  VehicleID/1 -> MATLAB Function1/2(VehicleID)
  Pilot/1 -> OFDM Modulator1/2

== system a2024_V2X_6V_Simulink_model/Vehicle 3 ==
  trigger : Inport
  busActors3Test1 : Inport  Port=2
  Pilot : Inport  Port=3
  VehicleID : Inport  Port=4
  Constant3 : Constant  Value=[zeros(19,1)']  SampleTime=-1
  Entity Multicast2 : EntityMulticast  InputPortMessageModes=m
  Integer to Bit Converter3 : simulink/Logic and Bit Operations/Integer to Bit Converter  nbits=16  signedInputValues=Signed  bitOrder=MSB first  outDtype=boolean
  MATLAB Function2 : MATLAB Function  TreatAsAtomicUnit=on
  OFDM Modulator2 : commofdm/OFDM Modulator  StatePerturbationForJacobian=1.0e-05  FFTLength=64  NumGuardBandCarriers=[0;0]  InsertDCNull=on  PilotInputPort=on  PilotCarrierIndices=[12; 26; 40; 54]  CyclicPrefixLength=32  Windowing=off  WindowLength=16  OversamplingFactor=3  NumSymbols=1  NumTransmitAntennas=1  SimulateUsing=Interpreted execution
  Rectangular QAM Modulator Baseband3 : commdigbbndam3/Rectangular QAM Modulator Baseband  M=2^6  InType=Bit  Enc=Binary  Mapping=[0:15]  PowType=Average Power  MinDist=2  AvgPow=P_Signal  PeakPow=1  Ph=0  outDtype=double  outWordLen=16  outUDDataType=sfix(16)  outFracLenMode=Best precision  outFracLen=15  outDataTypeStr=double  outLastDataTypeStr=double
      settings: LibrarySourceBlock=|
      | commhdldigbbndam/Rectangular QAM
      | Modulator
      | Baseband
  Send2 : Send  OutputPortMessageModes=m
  Vector Concatenate2 : Concatenate
  wires:
  MATLAB Function2/1(intVector) -> Integer to Bit Converter3/1
  OFDM Modulator2/1 -> Send2/1  "OFDM modulated"
  busActors3Test1/1 -> MATLAB Function2/1(busActors3Test1)
  Vector Concatenate2/1 -> OFDM Modulator2/1  "After QAM Mod"
  Send2/1 -> Entity Multicast2/1
  Integer to Bit Converter3/1 -> Rectangular QAM Modulator Baseband3/1
  Rectangular QAM Modulator Baseband3/1 -> Vector Concatenate2/1
  Pilot/1 -> OFDM Modulator2/2
  Constant3/1 -> Vector Concatenate2/2
  VehicleID/1 -> MATLAB Function2/2(VehicleID)
  trigger/1 -> MATLAB Function2/Trigger

== system a2024_V2X_6V_Simulink_model/Calculate PDR/PDR V1 ==
  Sent packet : Inport
  Received packets : Inport  Port=2
  Vehicle ID : Inport  Port=3
  Add : Sum  Commented=on  Inputs=-+
  Bus Selector3 : BusSelector  Commented=on  OutputSignals=ActorID,Position,Velocity,Roll,Pitch,Yaw,AngularVelocity
  Constant : Constant  Commented=on
  Data Type Conversion1 : DataTypeConversion  Commented=on  OutDataTypeStr=double  SaturateOnIntegerOverflow=off  RndMeth=Floor
  MATLAB Function : MATLAB Function  TreatAsAtomicUnit=on
  MATLAB Function1 : MATLAB Function  TreatAsAtomicUnit=on
  MATLAB Function2 : MATLAB Function  TreatAsAtomicUnit=on
  MATLAB Function6 : MATLAB Function  Commented=on  TreatAsAtomicUnit=on
  Matrix Concatenate : Concatenate  Mode=Multidimensional array  ConcatenateDimension=2
  Round : Rounding  Commented=on  Operator=round
  Selector : Selector  Commented=through  IndexOptions=Starting index (dialog)  Indices=3  OutputSizes=13
  Transpose : Math  Commented=on  Operator=transpose
  Vector Concatenate1 : Concatenate  Commented=on  NumInputs=7
  PDR1 : Outport
  Vectors output : Outport  Port=2
  wires:
  MATLAB Function2/1(y) -> Selector/1
  Received packets/1 -> MATLAB Function2/2(u)
  MATLAB Function1/1(y) -> Matrix Concatenate/1, MATLAB Function/1(Tx)
  MATLAB Function/1(PDR) -> PDR1/1
  Matrix Concatenate/1 -> Vectors output/1
  Selector/1 -> MATLAB Function/2(Rx), Matrix Concatenate/2
  Vehicle ID/1 -> MATLAB Function1/2(Vehicle_ID), MATLAB Function2/1(Vehicle_ID)
  ? -> MATLAB Function6/2(vehicleID)
  Bus Selector3/6 -> Vector Concatenate1/6  "<Yaw>"
  Bus Selector3/4 -> Vector Concatenate1/4  "<Roll>"
  Constant/1 -> Add/1
  Bus Selector3/7 -> Vector Concatenate1/7  "<AngularVelocity>"
  Vector Concatenate1/1 -> Transpose/1
  Add/1 -> Vector Concatenate1/1
  MATLAB Function6/1(y) -> Bus Selector3/1
  Bus Selector3/3 -> Vector Concatenate1/3  "<Velocity>"
  Bus Selector3/2 -> Vector Concatenate1/2  "<Position>"
  ? -> MATLAB Function6/1(u)
  Bus Selector3/5 -> Vector Concatenate1/5  "<Pitch>"
  Bus Selector3/1 -> Add/2  "<ActorID>"
  Transpose/1 -> Round/1
  Round/1 -> Data Type Conversion1/1
  Sent packet/1 -> MATLAB Function1/1(u)

== system a2024_V2X_6V_Simulink_model/Calculate PDR/PDR V2 ==
  Sent packet : Inport
  Received packets : Inport  Port=2
  Vehicle ID : Inport  Port=3
  Add : Sum  Commented=on  Inputs=-+
  Bus Selector3 : BusSelector  Commented=on  OutputSignals=ActorID,Position,Velocity,Roll,Pitch,Yaw,AngularVelocity
  Constant : Constant  Commented=on
  Data Type Conversion1 : DataTypeConversion  Commented=on  OutDataTypeStr=double  SaturateOnIntegerOverflow=off  RndMeth=Floor
  MATLAB Function : MATLAB Function  TreatAsAtomicUnit=on
  MATLAB Function1 : MATLAB Function  TreatAsAtomicUnit=on
  MATLAB Function2 : MATLAB Function  TreatAsAtomicUnit=on
  MATLAB Function6 : MATLAB Function  Commented=on  TreatAsAtomicUnit=on
  Matrix Concatenate : Concatenate  Mode=Multidimensional array  ConcatenateDimension=2
  Round : Rounding  Commented=on  Operator=round
  Selector : Selector  Commented=through  IndexOptions=Starting index (dialog)  Indices=3  OutputSizes=13
  Transpose : Math  Commented=on  Operator=transpose
  Vector Concatenate1 : Concatenate  Commented=on  NumInputs=7
  PDR1 : Outport
  Vectors output : Outport  Port=2
  wires:
  Sent packet/1 -> MATLAB Function1/1(u)
  Round/1 -> Data Type Conversion1/1
  Transpose/1 -> Round/1
  Bus Selector3/1 -> Add/2  "<ActorID>"
  Bus Selector3/5 -> Vector Concatenate1/5  "<Pitch>"
  ? -> MATLAB Function6/1(u)
  Bus Selector3/2 -> Vector Concatenate1/2  "<Position>"
  Bus Selector3/3 -> Vector Concatenate1/3  "<Velocity>"
  MATLAB Function6/1(y) -> Bus Selector3/1
  Add/1 -> Vector Concatenate1/1
  Vector Concatenate1/1 -> Transpose/1
  Bus Selector3/7 -> Vector Concatenate1/7  "<AngularVelocity>"
  Constant/1 -> Add/1
  Bus Selector3/4 -> Vector Concatenate1/4  "<Roll>"
  Bus Selector3/6 -> Vector Concatenate1/6  "<Yaw>"
  ? -> MATLAB Function6/2(vehicleID)
  Vehicle ID/1 -> MATLAB Function2/1(Vehicle_ID), MATLAB Function1/2(Vehicle_ID)
  Selector/1 -> Matrix Concatenate/2, MATLAB Function/2(Rx)
  Matrix Concatenate/1 -> Vectors output/1
  MATLAB Function/1(PDR) -> PDR1/1
  MATLAB Function1/1(y) -> MATLAB Function/1(Tx), Matrix Concatenate/1
  Received packets/1 -> MATLAB Function2/2(u)
  MATLAB Function2/1(y) -> Selector/1

== system a2024_V2X_6V_Simulink_model/Calculate PDR/PDR V3 ==
  Sent packet : Inport
  Received packets : Inport  Port=2
  Vehicle ID : Inport  Port=3
  Add : Sum  Commented=on  Inputs=-+
  Bus Selector3 : BusSelector  Commented=on  OutputSignals=ActorID,Position,Velocity,Roll,Pitch,Yaw,AngularVelocity
  Constant : Constant  Commented=on
  Data Type Conversion1 : DataTypeConversion  Commented=on  OutDataTypeStr=double  SaturateOnIntegerOverflow=off  RndMeth=Floor
  MATLAB Function : MATLAB Function  TreatAsAtomicUnit=on
  MATLAB Function1 : MATLAB Function  TreatAsAtomicUnit=on
  MATLAB Function2 : MATLAB Function  TreatAsAtomicUnit=on
  MATLAB Function6 : MATLAB Function  Commented=on  TreatAsAtomicUnit=on
  Matrix Concatenate : Concatenate  Mode=Multidimensional array  ConcatenateDimension=2
  Round : Rounding  Commented=on  Operator=round
  Selector : Selector  Commented=through  IndexOptions=Starting index (dialog)  Indices=3  OutputSizes=13
  Transpose : Math  Commented=on  Operator=transpose
  Vector Concatenate1 : Concatenate  Commented=on  NumInputs=7
  PDR1 : Outport
  Vectors output : Outport  Port=2
  wires:
  MATLAB Function2/1(y) -> Selector/1
  Received packets/1 -> MATLAB Function2/2(u)
  MATLAB Function1/1(y) -> Matrix Concatenate/1, MATLAB Function/1(Tx)
  MATLAB Function/1(PDR) -> PDR1/1
  Matrix Concatenate/1 -> Vectors output/1
  Selector/1 -> MATLAB Function/2(Rx), Matrix Concatenate/2
  Vehicle ID/1 -> MATLAB Function1/2(Vehicle_ID), MATLAB Function2/1(Vehicle_ID)
  ? -> MATLAB Function6/2(vehicleID)
  Bus Selector3/6 -> Vector Concatenate1/6  "<Yaw>"
  Bus Selector3/4 -> Vector Concatenate1/4  "<Roll>"
  Constant/1 -> Add/1
  Bus Selector3/7 -> Vector Concatenate1/7  "<AngularVelocity>"
  Vector Concatenate1/1 -> Transpose/1
  Add/1 -> Vector Concatenate1/1
  MATLAB Function6/1(y) -> Bus Selector3/1
  Bus Selector3/3 -> Vector Concatenate1/3  "<Velocity>"
  Bus Selector3/2 -> Vector Concatenate1/2  "<Position>"
  ? -> MATLAB Function6/1(u)
  Bus Selector3/5 -> Vector Concatenate1/5  "<Pitch>"
  Bus Selector3/1 -> Add/2  "<ActorID>"
  Transpose/1 -> Round/1
  Round/1 -> Data Type Conversion1/1
  Sent packet/1 -> MATLAB Function1/1(u)

== system a2024_V2X_6V_Simulink_model/Calculate PDR/PDR V4 ==
  Sent packet : Inport
  Received packets : Inport  Port=2
  Vehicle ID : Inport  Port=3
  Add : Sum  Commented=on  Inputs=-+
  Bus Selector3 : BusSelector  Commented=on  OutputSignals=ActorID,Position,Velocity,Roll,Pitch,Yaw,AngularVelocity
  Constant : Constant  Commented=on
  Data Type Conversion1 : DataTypeConversion  Commented=on  OutDataTypeStr=double  SaturateOnIntegerOverflow=off  RndMeth=Floor
  MATLAB Function : MATLAB Function  TreatAsAtomicUnit=on
  MATLAB Function1 : MATLAB Function  TreatAsAtomicUnit=on
  MATLAB Function2 : MATLAB Function  TreatAsAtomicUnit=on
  MATLAB Function6 : MATLAB Function  Commented=on  TreatAsAtomicUnit=on
  Matrix Concatenate : Concatenate  Mode=Multidimensional array  ConcatenateDimension=2
  Round : Rounding  Commented=on  Operator=round
  Selector : Selector  Commented=through  IndexOptions=Starting index (dialog)  Indices=3  OutputSizes=13
  Transpose : Math  Commented=on  Operator=transpose
  Vector Concatenate1 : Concatenate  Commented=on  NumInputs=7
  PDR1 : Outport
  Vectors output : Outport  Port=2
  wires:
  Sent packet/1 -> MATLAB Function1/1(u)
  Round/1 -> Data Type Conversion1/1
  Transpose/1 -> Round/1
  Bus Selector3/1 -> Add/2  "<ActorID>"
  Bus Selector3/5 -> Vector Concatenate1/5  "<Pitch>"
  ? -> MATLAB Function6/1(u)
  Bus Selector3/2 -> Vector Concatenate1/2  "<Position>"
  Bus Selector3/3 -> Vector Concatenate1/3  "<Velocity>"
  MATLAB Function6/1(y) -> Bus Selector3/1
  Add/1 -> Vector Concatenate1/1
  Vector Concatenate1/1 -> Transpose/1
  Bus Selector3/7 -> Vector Concatenate1/7  "<AngularVelocity>"
  Constant/1 -> Add/1
  Bus Selector3/4 -> Vector Concatenate1/4  "<Roll>"
  Bus Selector3/6 -> Vector Concatenate1/6  "<Yaw>"
  ? -> MATLAB Function6/2(vehicleID)
  Vehicle ID/1 -> MATLAB Function2/1(Vehicle_ID), MATLAB Function1/2(Vehicle_ID)
  Selector/1 -> Matrix Concatenate/2, MATLAB Function/2(Rx)
  Matrix Concatenate/1 -> Vectors output/1
  MATLAB Function/1(PDR) -> PDR1/1
  MATLAB Function1/1(y) -> MATLAB Function/1(Tx), Matrix Concatenate/1
  Received packets/1 -> MATLAB Function2/2(u)
  MATLAB Function2/1(y) -> Selector/1

== system a2024_V2X_6V_Simulink_model/Calculate PDR/PDR V5 ==
  Sent packet : Inport
  Received packets : Inport  Port=2
  Vehicle ID : Inport  Port=3
  Add : Sum  Commented=on  Inputs=-+
  Bus Selector3 : BusSelector  Commented=on  OutputSignals=ActorID,Position,Velocity,Roll,Pitch,Yaw,AngularVelocity
  Constant : Constant  Commented=on
  Data Type Conversion1 : DataTypeConversion  Commented=on  OutDataTypeStr=double  SaturateOnIntegerOverflow=off  RndMeth=Floor
  MATLAB Function : MATLAB Function  TreatAsAtomicUnit=on
  MATLAB Function1 : MATLAB Function  TreatAsAtomicUnit=on
  MATLAB Function2 : MATLAB Function  TreatAsAtomicUnit=on
  MATLAB Function6 : MATLAB Function  Commented=on  TreatAsAtomicUnit=on
  Matrix Concatenate : Concatenate  Mode=Multidimensional array  ConcatenateDimension=2
  Round : Rounding  Commented=on  Operator=round
  Selector : Selector  Commented=through  IndexOptions=Starting index (dialog)  Indices=3  OutputSizes=13
  Transpose : Math  Commented=on  Operator=transpose
  Vector Concatenate1 : Concatenate  Commented=on  NumInputs=7
  PDR1 : Outport
  Vectors output : Outport  Port=2
  wires:
  MATLAB Function2/1(y) -> Selector/1
  Received packets/1 -> MATLAB Function2/2(u)
  MATLAB Function1/1(y) -> Matrix Concatenate/1, MATLAB Function/1(Tx)
  MATLAB Function/1(PDR) -> PDR1/1
  Matrix Concatenate/1 -> Vectors output/1
  Selector/1 -> MATLAB Function/2(Rx), Matrix Concatenate/2
  Vehicle ID/1 -> MATLAB Function1/2(Vehicle_ID), MATLAB Function2/1(Vehicle_ID)
  ? -> MATLAB Function6/2(vehicleID)
  Bus Selector3/6 -> Vector Concatenate1/6  "<Yaw>"
  Bus Selector3/4 -> Vector Concatenate1/4  "<Roll>"
  Constant/1 -> Add/1
  Bus Selector3/7 -> Vector Concatenate1/7  "<AngularVelocity>"
  Vector Concatenate1/1 -> Transpose/1
  Add/1 -> Vector Concatenate1/1
  MATLAB Function6/1(y) -> Bus Selector3/1
  Bus Selector3/3 -> Vector Concatenate1/3  "<Velocity>"
  Bus Selector3/2 -> Vector Concatenate1/2  "<Position>"
  ? -> MATLAB Function6/1(u)
  Bus Selector3/5 -> Vector Concatenate1/5  "<Pitch>"
  Bus Selector3/1 -> Add/2  "<ActorID>"
  Transpose/1 -> Round/1
  Round/1 -> Data Type Conversion1/1
  Sent packet/1 -> MATLAB Function1/1(u)

== system a2024_V2X_6V_Simulink_model/Calculate PDR/PDR V6 ==
  Sent packet : Inport
  Received packets : Inport  Port=2
  Vehicle ID : Inport  Port=3
  Add : Sum  Commented=on  Inputs=-+
  Bus Selector3 : BusSelector  Commented=on  OutputSignals=ActorID,Position,Velocity,Roll,Pitch,Yaw,AngularVelocity
  Constant : Constant  Commented=on
  Data Type Conversion1 : DataTypeConversion  Commented=on  OutDataTypeStr=double  SaturateOnIntegerOverflow=off  RndMeth=Floor
  MATLAB Function : MATLAB Function  TreatAsAtomicUnit=on
  MATLAB Function1 : MATLAB Function  TreatAsAtomicUnit=on
  MATLAB Function2 : MATLAB Function  TreatAsAtomicUnit=on
  MATLAB Function6 : MATLAB Function  Commented=on  TreatAsAtomicUnit=on
  Matrix Concatenate : Concatenate  Mode=Multidimensional array  ConcatenateDimension=2
  Round : Rounding  Commented=on  Operator=round
  Selector : Selector  Commented=through  IndexOptions=Starting index (dialog)  Indices=3  OutputSizes=13
  Transpose : Math  Commented=on  Operator=transpose
  Vector Concatenate1 : Concatenate  Commented=on  NumInputs=7
  PDR1 : Outport
  Vectors output : Outport  Port=2
  wires:
  Sent packet/1 -> MATLAB Function1/1(u)
  Round/1 -> Data Type Conversion1/1
  Transpose/1 -> Round/1
  Bus Selector3/1 -> Add/2  "<ActorID>"
  Bus Selector3/5 -> Vector Concatenate1/5  "<Pitch>"
  ? -> MATLAB Function6/1(u)
  Bus Selector3/2 -> Vector Concatenate1/2  "<Position>"
  Bus Selector3/3 -> Vector Concatenate1/3  "<Velocity>"
  MATLAB Function6/1(y) -> Bus Selector3/1
  Add/1 -> Vector Concatenate1/1
  Vector Concatenate1/1 -> Transpose/1
  Bus Selector3/7 -> Vector Concatenate1/7  "<AngularVelocity>"
  Constant/1 -> Add/1
  Bus Selector3/4 -> Vector Concatenate1/4  "<Roll>"
  Bus Selector3/6 -> Vector Concatenate1/6  "<Yaw>"
  ? -> MATLAB Function6/2(vehicleID)
  Vehicle ID/1 -> MATLAB Function2/1(Vehicle_ID), MATLAB Function1/2(Vehicle_ID)
  Selector/1 -> Matrix Concatenate/2, MATLAB Function/2(Rx)
  Matrix Concatenate/1 -> Vectors output/1
  MATLAB Function/1(PDR) -> PDR1/1
  MATLAB Function1/1(y) -> MATLAB Function/1(Tx), Matrix Concatenate/1
  Received packets/1 -> MATLAB Function2/2(u)
  MATLAB Function2/1(y) -> Selector/1

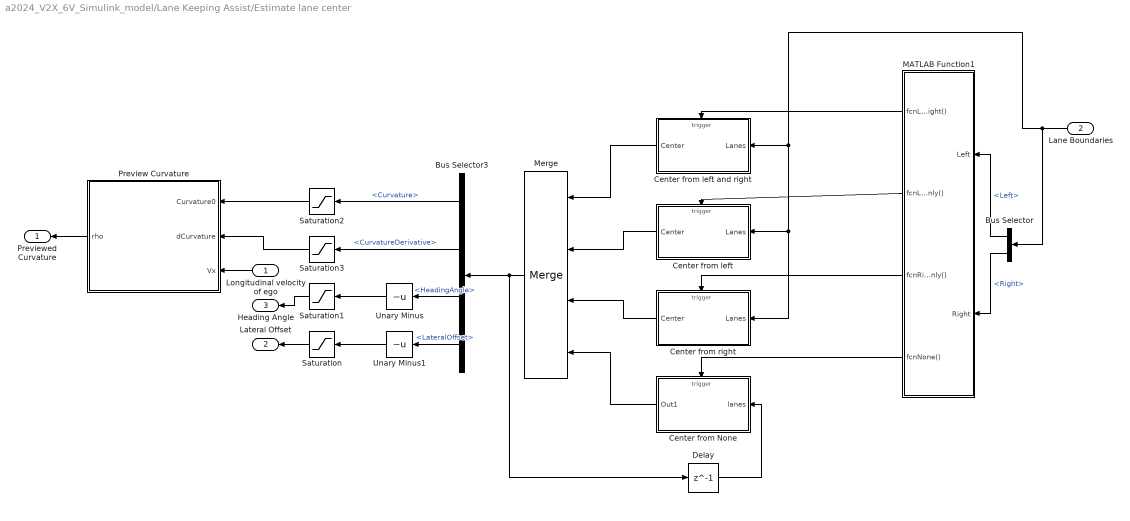
== system a2024_V2X_6V_Simulink_model/Lane Keeping Assist/Estimate lane center ==
  Longitudinal velocity of ego : Inport
  Lane Boundaries : Inport  Port=2
  Bus Selector : BusSelector  OutputSignals=Left,Right
  Bus Selector3 : BusSelector  OutputSignals=Curvature,CurvatureDerivative,HeadingAngle,LateralOffset
  Center from None : Subsystem
  Center from left : Subsystem
  Center from left and right : Subsystem
  Center from right : Subsystem
  Delay : Delay  DelayLength=1
  MATLAB Function1 : MATLAB Function  TreatAsAtomicUnit=on
  Merge : Merge  Inputs=4  InputPortOffsets=4
  Preview Curvature : MATLAB Function  TreatAsAtomicUnit=on  SystemSampleTime=Ts
  Saturation : Saturate
  Saturation1 : Saturate  UpperLimit=0.6  LowerLimit=-0.6
  Saturation2 : Saturate  UpperLimit=0.15  LowerLimit=-0.15
  Saturation3 : Saturate  UpperLimit=0.06  LowerLimit=-0.06
  Unary Minus : UnaryMinus
  Unary Minus1 : UnaryMinus
  Previewed Curvature : Outport
  Lateral Offset : Outport  Port=2
  Heading Angle : Outport  Port=3
  wires:
  Bus Selector3/1 -> Saturation2/1  "<Curvature>"
  Bus Selector3/2 -> Saturation3/1  "<CurvatureDerivative>"
  Bus Selector3/4 -> Unary Minus1/1  "<LateralOffset>"
  Saturation1/1 -> Heading Angle/1
  Bus Selector3/3 -> Unary Minus/1  "<HeadingAngle>"
  MATLAB Function1/1(fcnLeftAndRight()) -> Center from left and right/Trigger
  MATLAB Function1/2(fcnLeftOnly()) -> Center from left/Trigger
  Saturation3/1 -> Preview Curvature/2(dCurvature)
  MATLAB Function1/3(fcnRightOnly()) -> Center from right/Trigger
  Unary Minus/1 -> Saturation1/1
  Delay/1 -> Center from None/1(lanes)
  MATLAB Function1/4(fcnNone()) -> Center from None/Trigger
  Saturation2/1 -> Preview Curvature/1(Curvature0)
  Unary Minus1/1 -> Saturation/1
  Preview Curvature/1(rho) -> Previewed Curvature/1
  Saturation/1 -> Lateral Offset/1
  Longitudinal velocity of ego/1 -> Preview Curvature/3(Vx)
  Lane Boundaries/1 -> Bus Selector/1, Center from left/1(Lanes), Center from right/1(Lanes), Center from left and right/1(Lanes)
  Bus Selector/1 -> MATLAB Function1/1(Left)  "<Left>"
  Bus Selector/2 -> MATLAB Function1/2(Right)  "<Right>"
  Center from None/1(Out1) -> Merge/4
  Center from left and right/1(Center) -> Merge/1
  Center from right/1(Center) -> Merge/3
  Center from left/1(Center) -> Merge/2
  Merge/1 -> Delay/1, Bus Selector3/1

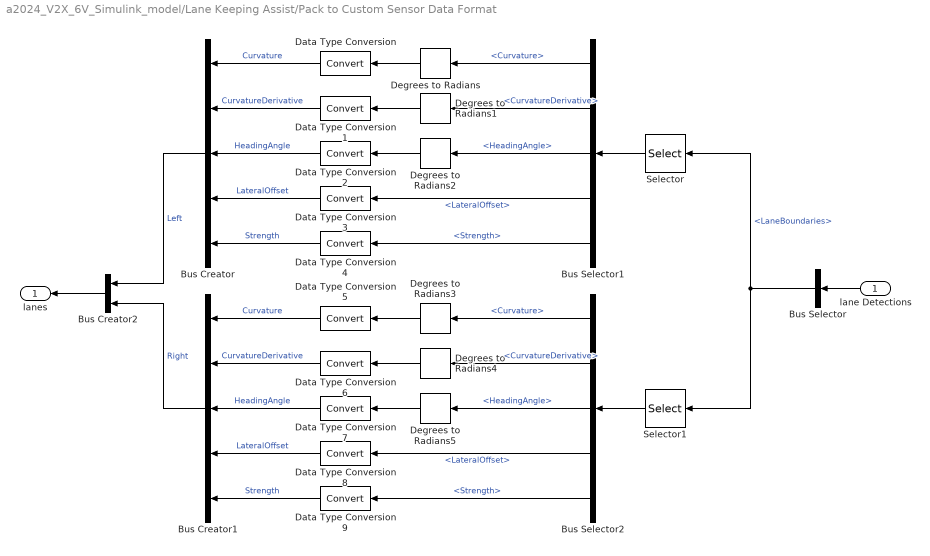
== system a2024_V2X_6V_Simulink_model/Lane Keeping Assist/Pack to Custom Sensor Data Format ==
  lane Detections : Inport
  Bus Creator : BusCreator  Inputs=5
  Bus Creator1 : BusCreator  Inputs=5
  Bus Creator2 : BusCreator  Inputs=2
  Bus Selector : BusSelector  OutputSignals=LaneBoundaries
  Bus Selector1 : BusSelector  OutputSignals=Curvature,CurvatureDerivative,HeadingAngle,LateralOffset,Strength
  Bus Selector2 : BusSelector  OutputSignals=Curvature,CurvatureDerivative,HeadingAngle,LateralOffset,Strength
  Data Type Conversion{,1..9} (10 alike) : DataTypeConversion  SaturateOnIntegerOverflow=off  RndMeth=Floor
  Degrees to Radians{,1..5} (6 alike) : simulink_extras/Transformations/Degrees to Radians
  Selector : Selector  IndexMode=Zero-based  InputPortWidth=30  IndexOptions=Index vector (dialog)  Indices=1  OutputSizes=1
  Selector1 : Selector  InputPortWidth=30  IndexOptions=Index vector (dialog)  Indices=2  OutputSizes=1
  lanes : Outport  VectorParamsAs1DForOutWhenUnconnected=off
  wires:
  lane Detections/1 -> Bus Selector/1
  Bus Selector/1 -> Selector/1, Selector1/1  "<LaneBoundaries>"
  Selector/1 -> Bus Selector1/1
  Bus Selector1/2 -> Degrees to Radians1/1  "<CurvatureDerivative>"
  Bus Selector1/1 -> Degrees to Radians/1  "<Curvature>"
  Bus Selector1/3 -> Degrees to Radians2/1  "<HeadingAngle>"
  Degrees to Radians/1 -> Data Type Conversion/1
  Degrees to Radians1/1 -> Data Type Conversion1/1
  Degrees to Radians2/1 -> Data Type Conversion2/1
  Bus Selector1/4 -> Data Type Conversion3/1  "<LateralOffset>"
  Bus Selector1/5 -> Data Type Conversion4/1  "<Strength>"
  Data Type Conversion/1 -> Bus Creator/1  "Curvature"
  Data Type Conversion1/1 -> Bus Creator/2  "CurvatureDerivative"
  Data Type Conversion2/1 -> Bus Creator/3  "HeadingAngle"
  Data Type Conversion3/1 -> Bus Creator/4  "LateralOffset"
  Data Type Conversion4/1 -> Bus Creator/5  "Strength"
  Data Type Conversion9/1 -> Bus Creator1/5  "Strength"
  Data Type Conversion6/1 -> Bus Creator1/2  "CurvatureDerivative"
  Data Type Conversion7/1 -> Bus Creator1/3  "HeadingAngle"
  Data Type Conversion8/1 -> Bus Creator1/4  "LateralOffset"
  Data Type Conversion5/1 -> Bus Creator1/1  "Curvature"
  Bus Selector2/1 -> Degrees to Radians3/1  "<Curvature>"
  Selector1/1 -> Bus Selector2/1
  Bus Selector2/4 -> Data Type Conversion8/1  "<LateralOffset>"
  Bus Selector2/5 -> Data Type Conversion9/1  "<Strength>"
  Bus Selector2/2 -> Degrees to Radians4/1  "<CurvatureDerivative>"
  Degrees to Radians5/1 -> Data Type Conversion7/1
  Degrees to Radians3/1 -> Data Type Conversion5/1
  Degrees to Radians4/1 -> Data Type Conversion6/1
  Bus Selector2/3 -> Degrees to Radians5/1  "<HeadingAngle>"
  Bus Creator2/1 -> lanes/1
  Bus Creator/1 -> Bus Creator2/1  "Left"
  Bus Creator1/1 -> Bus Creator2/2  "Right"

== system a2024_V2X_6V_Simulink_model/Lane Keeping Assist/Subsystem ==
  Lane Assist Offset : Inport
  Lane Sensor data : Inport  Port=2
  Bus Selector3 : BusSelector  OutputSignals=Left.LateralOffset,Right.LateralOffset
  Gain3 : Gain  Gain=-1
  Logical Operator : Logic  Operator=OR  AllPortsSameDT=off  OutDataTypeStr=boolean
  Relational Operator : RelationalOperator  Operator=<=  OutDataTypeStr=boolean  RndMeth=Simplest  InputSameDT=off
  Relational Operator1 : RelationalOperator  OutDataTypeStr=boolean  RndMeth=Simplest  InputSameDT=off
  Departure Detected : Outport
  wires:
  Relational Operator1/1 -> Logical Operator/2
  Bus Selector3/2 -> Relational Operator1/1  "<LateralOffset>"
  Bus Selector3/1 -> Relational Operator/1  "<LateralOffset>"
  Relational Operator/1 -> Logical Operator/1
  Logical Operator/1 -> Departure Detected/1
  Gain3/1 -> Relational Operator1/2
  Lane Assist Offset/1 -> Gain3/1, Relational Operator/2
  Lane Sensor data/1 -> Bus Selector3/1

== system a2024_V2X_6V_Simulink_model/Lane Keeping Assist/Subsystem2 ==
  Enable : Inport
  Set : Inport  Port=2
  Assisted Steer : Inport  Port=3
  Driver Steer : Inport  Port=4
  AND : Logic  IconShape=distinctive  AllPortsSameDT=off  OutDataTypeStr=boolean
  Latch Assist : Subsystem
  Subsystem1 : Subsystem
  Switch : Switch  Criteria=u2 > Threshold  SaturateOnIntegerOverflow=off  InputSameDT=off
  Status : Outport
  SteeringAngle in rad : Outport  Port=2
  wires:
  Enable/1 -> AND/1
  AND/1 -> Status/1, Switch/2
  Latch Assist/1(Assist) -> AND/2
  Subsystem1/1(Similar) -> Latch Assist/2(Reset)
  Driver Steer/1 -> Switch/3, Subsystem1/2(Driver Steer)
  Assisted Steer/1 -> Switch/1, Subsystem1/1(Assisted Steer)
  Switch/1 -> SteeringAngle in rad/1
  Set/1 -> Latch Assist/1(Set)

== system a2024_V2X_6V_Simulink_model/Queue/Switch Case Action Subsystem ==
  Actor1 : Inport
  Action Port : ActionPort  ActionPortLabel=case [ 0 ]:
  Out1 : Outport
  wires:
  Actor1/1 -> Out1/1

== system a2024_V2X_6V_Simulink_model/Queue/Switch Case Action Subsystem1 ==
  Actor1 : Inport
  Action Port : ActionPort  ActionPortLabel=case [ 1 ]:
  Out1 : Outport
  wires:
  Actor1/1 -> Out1/1

== system a2024_V2X_6V_Simulink_model/Queue/Switch Case Action Subsystem2 ==
  Actor1 : Inport
  Action Port : ActionPort  ActionPortLabel=case [ 2 ]:
  Out1 : Outport
  wires:
  Actor1/1 -> Out1/1

== system a2024_V2X_6V_Simulink_model/Queue/Switch Case Action Subsystem3 ==
  Actor1 : Inport
  Action Port : ActionPort  ActionPortLabel=case [ 3 ]:
  Out1 : Outport
  wires:
  Actor1/1 -> Out1/1

== system a2024_V2X_6V_Simulink_model/Queue/Switch Case Action Subsystem4 ==
  Actor1 : Inport
  Action Port : ActionPort  ActionPortLabel=case [ 4 ]:
  Out1 : Outport
  wires:
  Actor1/1 -> Out1/1

== system a2024_V2X_6V_Simulink_model/Queue/Switch Case Action Subsystem5 ==
  Actor1 : Inport
  Action Port : ActionPort  ActionPortLabel=case [ 5 ]:
  Out1 : Outport
  wires:
  Actor1/1 -> Out1/1
